simulink model "CL_Master_Runner_Test"  (R2020b)
settings: configuration reference "VLS_Standard_Configuration" (kept outside this file)
model workspace (MAT data in the model file):
  M_combineLogic = Simulink.Parameter
  M_combineLogic.Value = [0; 1; 0; 1]
  M_combineLogic.DataType = 'boolean'
  M_combineLogic.Dimensions = [4 1]
settings Model: DataDictionary=CL_MasterDD.sldd  EnableAccessToBaseWorkspace=off  Creator=mteama  LastModifiedBy=mtarek-a
settings ConfigSetRef: SourceName=VLS_Standard_Configuration

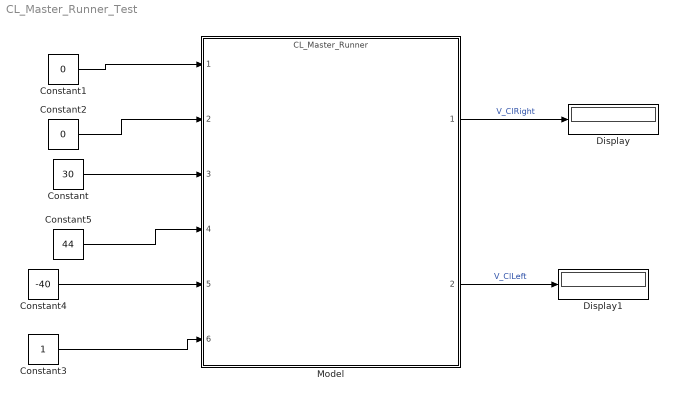
== system CL_Master_Runner_Test ==
  Constant : Constant  Value=30  OutDataTypeStr=fixdt(0,16,0.1,0)
  Constant1 : Constant  Value=0  OutDataTypeStr=boolean
  Constant2 : Constant  Value=0  OutDataTypeStr=boolean
  Constant3 : Constant  OutDataTypeStr=boolean
  Constant4 : Constant  Value=-40  OutDataTypeStr=fixdt(1,16,0.1,0)
  Constant5 : Constant  Value=44  OutDataTypeStr=fixdt(1,16,0.1,0)
  Display : Display
  Display1 : Display
  Model : ModelReference  ModelNameDialog=CL_Master_Runner.slx  SimulationMode=Normal  ModelReferenceVersion=7.12
  wires:
  Constant2/1 -> Model/2
  Constant1/1 -> Model/1
  Constant/1 -> Model/3
  Constant4/1 -> Model/5
  Constant5/1 -> Model/4
  Model/1 -> Display/1  "V_ClRight"
  Model/2 -> Display1/1  "V_ClLeft"
  Constant3/1 -> Model/6
